simulink model "Non_linear_sys"  (R2024b)
settings: Solver=VariableStepAuto  StartTime=0.0  StopTime=300  RelTol=1e-3
settings Model: Creator=shalh  LastModifiedBy=shalh

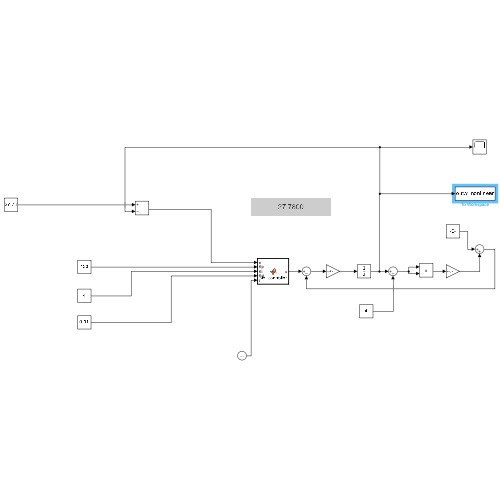
[thumbnail: Simulink's stored preview of the top-level diagram]
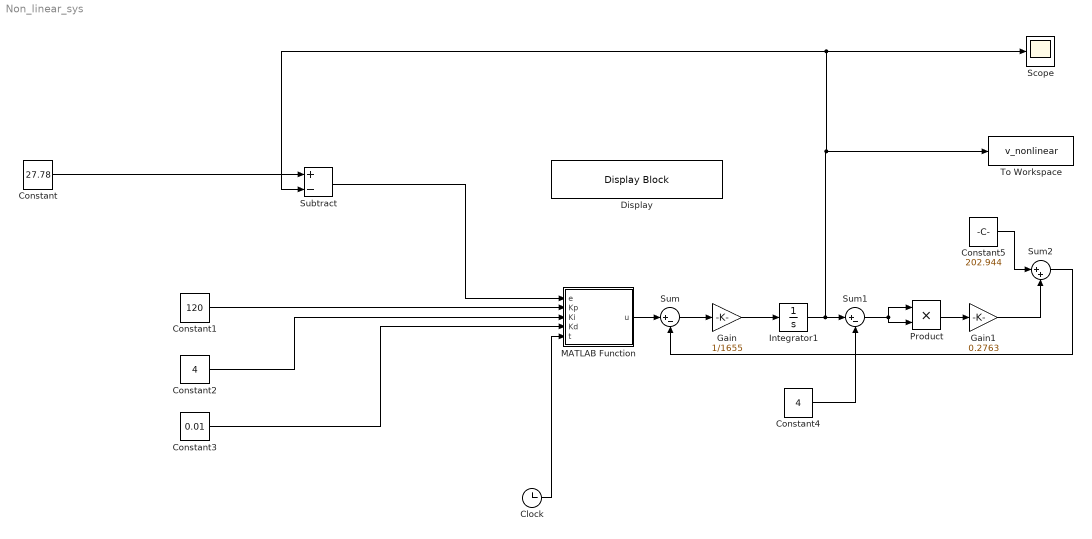
== system Non_linear_sys ==
  Clock : Clock
      settings: Decimation=40
  Constant : Constant  Value=27.78
  Constant1 : Constant  Value=120
  Constant2 : Constant  Value=4
  Constant3 : Constant  Value=0.01
  Constant4 : Constant  Value=4
  Constant5 : Constant  Value=202.944
  Display : DisplayBlock  LabelPosition=Hide  Transparency=1
  Gain : Gain  Gain=1/1655
  Gain1 : Gain  Gain=0.2763
  Integrator1 : Integrator
  MATLAB Function : MATLAB Function  TreatAsAtomicUnit=on
  Product : Product
  Scope : Scope
  Subtract : Sum  Inputs=+-
  Sum : Sum  Inputs=|+-
  Sum1 : Sum  Inputs=|+-
  Sum2 : Sum  Inputs=|++
  To Workspace : ToWorkspace  VariableName=v_nonlinear  SampleTime=-1
  wires:
  Product/1 -> Gain1/1
  Gain/1 -> Integrator1/1
  Sum/1 -> Gain/1
  Constant1/1 -> MATLAB Function/2(Kp)
  Constant4/1 -> Sum1/2
  Constant5/1 -> Sum2/1
  Integrator1/1 -> Subtract/2, Scope/1, To Workspace/1, Sum1/1
  Gain1/1 -> Sum2/2
  MATLAB Function/1(u) -> Sum/1
  Sum1/1 -> Product/2, Product/1
  Subtract/1 -> MATLAB Function/1(e)
  Clock/1 -> MATLAB Function/5(t)
  Sum2/1 -> Sum/2
  Constant2/1 -> MATLAB Function/3(Ki)
  Constant3/1 -> MATLAB Function/4(Kd)
  Constant/1 -> Subtract/1

== matlab function Non_linear_sys/MATLAB Function ==
  settings: updateMethod=DISCRETE
  data: e input double; Kp input; Ki input; Kd input; u output double; t input
function u = pid_controller(e,Kp,Ki, Kd, t)
  
    persistent e_integral e_prev t_prev
    if isempty(e_integral)
        e_integral = 0;
        e_prev = 0;
        t_prev = 0;
    end
    
    
    if t_prev == 0
        dt = 0.01; 
    else
        dt = t - t_prev;
    end
    
    e_integral = e_integral + e * dt;
    
    if dt > 0
        e_derivative = (e - e_prev) / dt;
    else
        e_derivative = 0;
    end
    
    u = Kp * e + Ki * e_integral + Kd * e_derivative;
    
    e_prev = e;
    disp(e);
    t_prev = t;
end
